simulink model "Beobachter_1D_Model"  (R2016b)
settings: Solver=VariableStepAuto  StartTime=0.0  StopTime=10.0  RelTol=1e-3
values from neighbouring files (symbols this model uses):
  A = [0, 1, 0; (m*g*l_C)/I_G, (-C_phi-C_psi)/I_G, C_psi/I_G; 0, C_psi/I_R, -C_psi/I_R]    [Beobachter_1D.m]    (also in Beobachter_1D_diskret.m)
  A_B = T_B\A*T_B    [Beobachter_1D.m]
  B = [0; -1/I_G; 1/I_R]    [Beobachter_1D.m]    (also in Beobachter_1D_diskret.m)
  B_B = T_B\B    [Beobachter_1D.m]
  C = [0, 1, 0]    [Beobachter_1D.m]    (also in Beobachter_1D_diskret.m = [0, 1, 0;0,0,1])
  C_B = C*T_B    [Beobachter_1D.m]
  k = lqr(A, B, Q, R)    [Beobachter_1D.m]    (also in Beobachter_1D_diskret.m = lqrd(A, B, Q, R, Ta))
  L = (a_B_soll - a_B_ist)'    [Beobachter_1D.m]
  T_B = [s_B, A*s_B, A^2*s_B]    [Beobachter_1D.m]
  x_0 = degtorad([5;0;0])    [Beobachter_1D_diskret.m]
  x_0_off = zeros(3,1)    [Beobachter_1D_diskret.m]
settings Model: Creator=michael  LastModifiedBy=michael

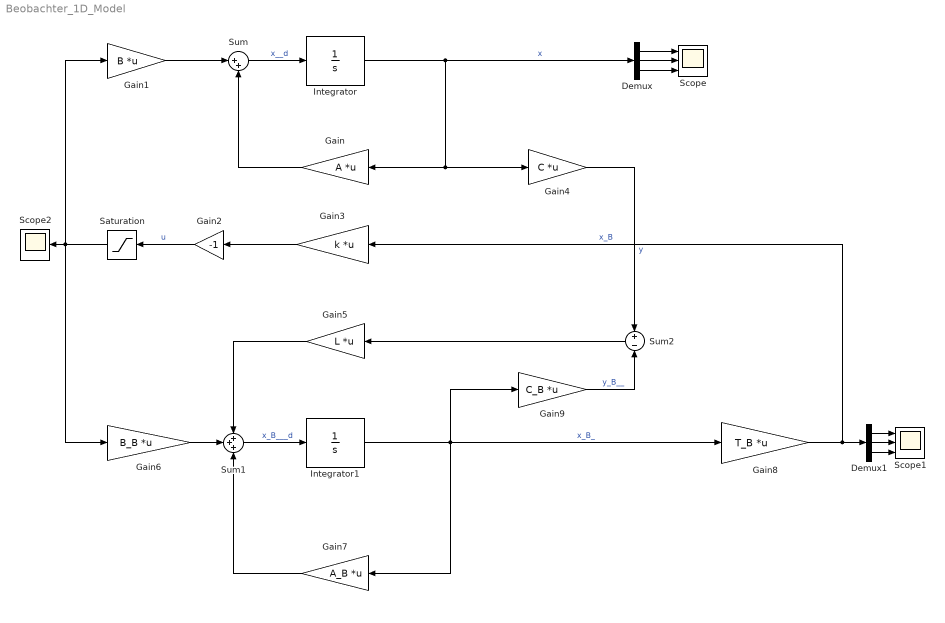
== system Beobachter_1D_Model ==
  Demux : Demux  Outputs=3
  Demux1 : Demux  Outputs=3
  Gain : Gain  Gain=A  Multiplication=Matrix(K*u) (u vector)
  Gain1 : Gain  Gain=B  Multiplication=Matrix(K*u) (u vector)
  Gain2 : Gain  Gain=-1
  Gain3 : Gain  Gain=k  Multiplication=Matrix(K*u) (u vector)
  Gain4 : Gain  Gain=C  Multiplication=Matrix(K*u) (u vector)
  Gain5 : Gain  Gain=L  Multiplication=Matrix(K*u) (u vector)
  Gain6 : Gain  Gain=B_B  Multiplication=Matrix(K*u) (u vector)
  Gain7 : Gain  Gain=A_B  Multiplication=Matrix(K*u) (u vector)
  Gain8 : Gain  Gain=T_B  Multiplication=Matrix(K*u) (u vector)
  Gain9 : Gain  Gain=C_B  Multiplication=Matrix(K*u) (u vector)
  Integrator : Integrator  InitialCondition=x_0
  Integrator1 : Integrator  InitialCondition=T_B\(x_0+x_0_off)
  Saturation : Saturate  UpperLimit=0.07  LowerLimit=-0.07
  Scope : Scope  NumInputPorts=3
  Scope1 : Scope  NumInputPorts=3
  Scope2 : Scope
  Sum : Sum  Inputs=|++
  Sum1 : Sum  Inputs=+++
  Sum2 : Sum  Inputs=+|-
  wires:
  Sum/1 -> Integrator/1  "x__d"
  Gain/1 -> Sum/2
  Gain1/1 -> Sum/1
  Gain2/1 -> Saturation/1  "u"
  Gain3/1 -> Gain2/1
  Integrator/1 -> Demux/1, Gain4/1, Gain/1  "x"
  Demux/1 -> Scope/1
  Demux/2 -> Scope/2
  Demux/3 -> Scope/3
  Gain4/1 -> Sum2/1  "y"
  Gain5/1 -> Sum1/1
  Gain6/1 -> Sum1/2
  Gain7/1 -> Sum1/3
  Sum1/1 -> Integrator1/1  "x_B___d"
  Integrator1/1 -> Gain9/1, Gain7/1, Gain8/1  "x_B_"
  Gain8/1 -> Gain3/1, Demux1/1  "x_B"
  Demux1/1 -> Scope1/1
  Demux1/2 -> Scope1/2
  Demux1/3 -> Scope1/3
  Sum2/1 -> Gain5/1
  Gain9/1 -> Sum2/2  "y_B__"
  Saturation/1 -> Scope2/1, Gain6/1, Gain1/1
